simulink model "problem4_diff_eq"  (R2020b)
settings: Solver=VariableStepAuto  StartTime=0.0  StopTime=10.0  RelTol=1e-3
settings Model: Creator=Gopinath Murugan  LastModifiedBy=Gopinath Murugan

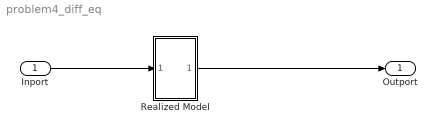
== system problem4_diff_eq ==
  Inport : Inport
  Realized Model : Subsystem
  Outport : Outport
  wires:
  Inport/1 -> Realized Model/1(In1)
  Realized Model/1(Out1) -> Outport/1

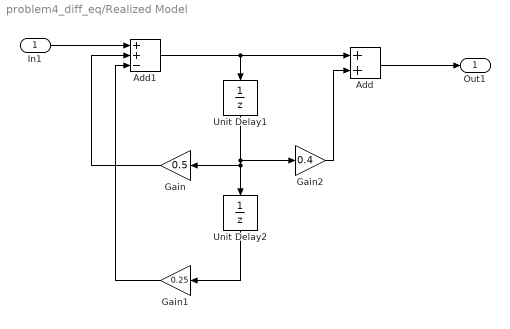
== system problem4_diff_eq/Realized Model ==
  In1 : Inport
  Add : Sum
  Add1 : Sum  Inputs=++-
  Gain : Gain  Gain=0.5
  Gain1 : Gain  Gain=0.25
  Gain2 : Gain  Gain=0.4
  Unit Delay1 : UnitDelay  SampleTime=-1  HasFrameUpgradeWarning=on
  Unit Delay2 : UnitDelay  SampleTime=-1  HasFrameUpgradeWarning=on
  Out1 : Outport
  wires:
  Gain1/1 -> Add1/3
  Unit Delay1/1 -> Gain/1, Unit Delay2/1, Gain2/1
  In1/1 -> Add1/1
  Add/1 -> Out1/1
  Add1/1 -> Add/1, Unit Delay1/1
  Gain2/1 -> Add/2
  Unit Delay2/1 -> Gain1/1
  Gain/1 -> Add1/2
